simulink model "cudemo_LiS_ECN_Model"  (R2016a)
settings: Solver=ode3  StartTime=0.0  StopTime=STOP_TIME  FixedStep=Ts  RelTol=1e-3
PreLoadFcn:
  | Ts = 1;
  | load cudemo_LiS_ECN_Model_nedc_BOP_2A
undefined symbols (not defined in the file or in its folder): DiscIntNeverNeededParam
libraries: LiS_ECN_Model_lib x1
settings Model: Creator=s220373  LastModifiedBy=e102261
settings DataIOCC: LimitDataPoints=on  SaveFormat=Array  SaveOutput=off  SignalLogging=off  DSMLogging=off  SaveTime=off
settings DebuggingCC: UnderspecifiedInitializationDetection=Classic  MergeDetectMultiDrivingBlocksExec=none  SolverPrmCheckMsg=warning
settings HardwareCC: ProdBitPerPointer=32  ProdLargestAtomicFloat=None  ProdIntDivRoundTo=Undefined  ProdEndianess=Unspecified  ProdWordSize=32  ProdHWDeviceType=32-bit Generic
settings ModelReferenceCC: PropagateSignalLabelsOutOfModel=off
settings ConfigComp: CovModelRefEnable=Off
settings ConfigurationSet: Description=SimMechanics 2G

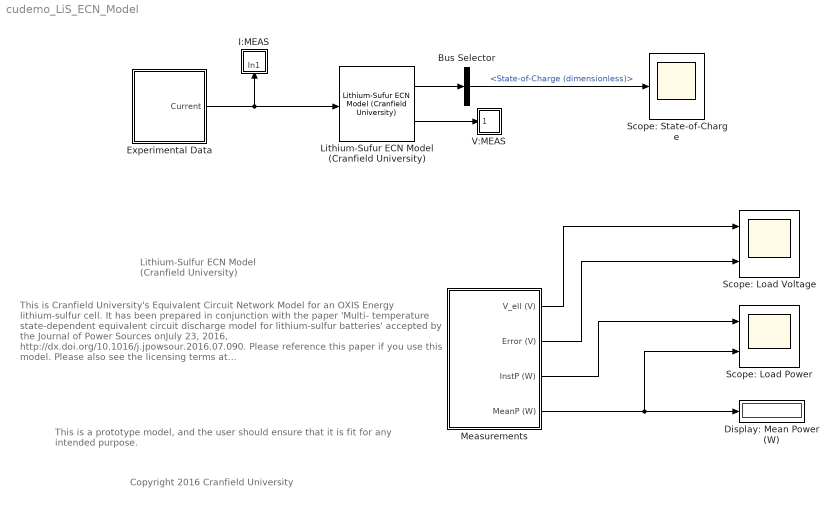
== system cudemo_LiS_ECN_Model ==
  note: Copyright 2016 Cranfield University
  note: This is Cranfield University's Equivalent Circuit Network Model for an OXIS Energy
      | lithium-sulfur cell. It has been prepared in conjunction with the paper 'Multi-
      | temperature state-dependent equivalent circuit discharge model for lithium-sulfur
      | batteries' accepted by the Journal of Power Sources onJuly 23, 2016,
      | http://dx.doi.org/10.1016/j.jpowsour.2016.07.090. Please reference this paper if
      | you use this model.
      |
      | Please also see the licensing terms at
      | http://dx.doi.org/10.17862/cranfield.rd.c.3292031
  note: Lithium-Sulfur ECN Model
      | (Cranfield University)
  note: This is a prototype model, and the user should ensure that it is fit for
      | any intended purpose.
  Bus Selector : BusSelector  OutputSignals=State-of-Charge (dimensionless)
  Display: Mean Power (W) : Display
  Experimental Data : Subsystem
  I:MEAS : Subsystem
  Lithium-Sufur ECN Model (Cranfield University) : LiS_ECN_Model_lib/Lithium-Sufur ECN Model (Cranfield University)  TempDegC=21  InitialSoC=1
      settings: AttributesFormatString=|
      | Temperature = %<TempDegC> deg C
      | Initial SoC = %<InitialSoC>
  Measurements : Subsystem
  Scope: Load Power : Scope  NumInputPorts=2
  Scope: Load Voltage : Scope  NumInputPorts=2
  Scope: State-of-Charge : Scope
  V:MEAS : Subsystem
  wires:
  Experimental Data/1(Current) -> Lithium-Sufur ECN Model (Cranfield University)/1, I:MEAS/1(In1)
  Lithium-Sufur ECN Model (Cranfield University)/2 -> V:MEAS/1(In1)
  Lithium-Sufur ECN Model (Cranfield University)/1 -> Bus Selector/1
  Bus Selector/1 -> Scope: State-of-Charge/1  "<State-of-Charge (dimensionless)>"
  Measurements/2(Error (V)) -> Scope: Load Voltage/2
  Measurements/3(InstP (W)) -> Scope: Load Power/1
  Measurements/1(V_ell (V)) -> Scope: Load Voltage/1
  Measurements/4(MeanP (W)) -> Scope: Load Power/2, Display: Mean Power (W)/1

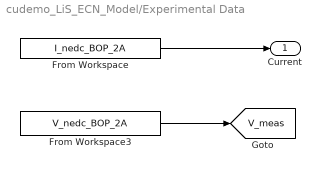
== system cudemo_LiS_ECN_Model/Experimental Data ==
  From Workspace : FromWorkspace  VariableName=I_nedc_BOP_2A  SampleTime=Ts  OutputAfterFinalValue=Setting to zero
  From Workspace3 : FromWorkspace  VariableName=V_nedc_BOP_2A  SampleTime=Ts  OutputAfterFinalValue=Holding final value
  Current : Outport  PortDimensions=1  SampleTime=Ts
  tag scope: V_meas=global
  wires:
  From Workspace/1 -> Current/1
  From Workspace3/1 -> [V_meas]

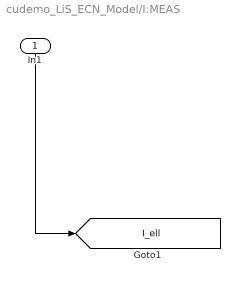
== system cudemo_LiS_ECN_Model/I:MEAS ==
  In1 : Inport
  tag scope: I_ell=global
  wires:
  In1/1 -> [I_ell]

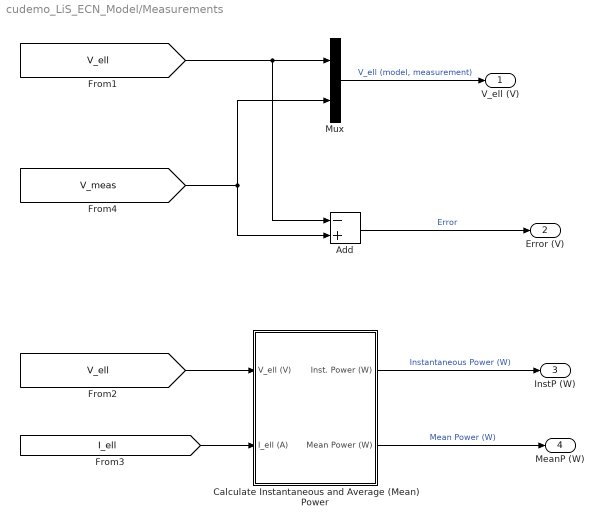
== system cudemo_LiS_ECN_Model/Measurements ==
  Add : Sum  Inputs=-+
  Calculate Instantaneous and Average (Mean) Power : Subsystem
  Mux : Mux  Inputs=2
  V_ell (V) : Outport
  Error (V) : Outport  Port=2
  InstP (W) : Outport  Port=3
  MeanP (W) : Outport  Port=4
  wires:
  [V_ell] -> Add/1, Mux/1
  [V_meas] -> Mux/2, Add/2
  Add/1 -> Error (V)/1  "Error"
  Mux/1 -> V_ell (V)/1  "V_ell (model, measurement)"
  [I_ell] -> Calculate Instantaneous and Average (Mean) Power/2(I_ell (A))
  Calculate Instantaneous and Average (Mean) Power/1(Inst. Power (W)) -> InstP (W)/1  "Instantaneous Power (W)"
  [V_ell] -> Calculate Instantaneous and Average (Mean) Power/1(V_ell (V))
  Calculate Instantaneous and Average (Mean) Power/2(Mean Power (W)) -> MeanP (W)/1  "Mean Power (W)"

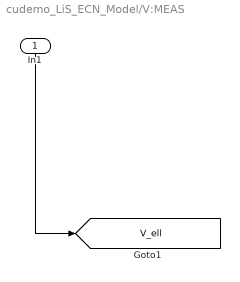
== system cudemo_LiS_ECN_Model/V:MEAS ==
  In1 : Inport
  tag scope: V_ell=global
  wires:
  In1/1 -> [V_ell]

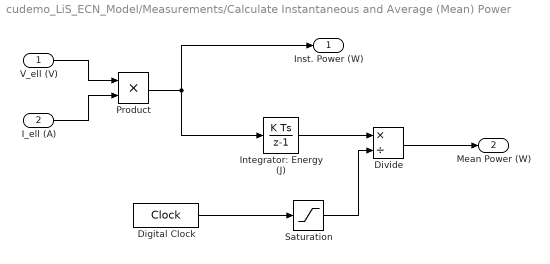
== system cudemo_LiS_ECN_Model/Measurements/Calculate Instantaneous and Average (Mean) Power ==
  V_ell (V) : Inport  PortDimensions=1  SampleTime=Ts
  I_ell (A) : Inport  Port=2  PortDimensions=1  SampleTime=Ts
  Digital Clock : DigitalClock  SampleTime=Ts
  Divide : Product  Inputs=*/
  Integrator: Energy (J) : DiscreteIntegrator  InitialConditionSetting=State (most efficient)  SampleTime=Ts  ICPrevOutput=DiscIntNeverNeededParam  ICPrevScaledInput=DiscIntNeverNeededParam
  Product : Product
  Saturation : Saturate  UpperLimit=inf  LowerLimit=Ts
  Inst. Power (W) : Outport
  Mean Power (W) : Outport  Port=2
  wires:
  Saturation/1 -> Divide/2
  V_ell (V)/1 -> Product/1
  I_ell (A)/1 -> Product/2
  Product/1 -> Inst. Power (W)/1, Integrator: Energy (J)/1
  Divide/1 -> Mean Power (W)/1
  Integrator: Energy (J)/1 -> Divide/1
  Digital Clock/1 -> Saturation/1
